simulink model "quadrotorsmodel1"  (R2025b)
settings: Solver=FixedStepAuto  StartTime=0.0  StopTime=SimulationTime  FixedStep=timestep  RelTol=1e-3
values from neighbouring files (symbols this model uses):
  g = 9.81    [TESA_Workspace1.m]    (also in TESA_Workspace2.m)
  I = eye(3,3)    [TESA_Workspace1.m]    (also in TESA_Workspace2.m)
  K = [1 1 1 1 ... (first row only)    [TESA_Workspace1.m]    (also in TESA_Workspace2.m)
  Kp = 1*Kp    [TESA_Workspace1.m]    (also in TESA_Workspace2.m)
  Kr = 1*Kr    [TESA_Workspace1.m]    (also in TESA_Workspace2.m)
  Kv = 1*Kv    [TESA_Workspace1.m]    (also in TESA_Workspace2.m)
  Kw = 1*Kw    [TESA_Workspace1.m]    (also in TESA_Workspace2.m)
  m = 4.34    [TESA_Workspace1.m]    (also in TESA_Workspace2.m)
settings Model: Creator=worap  LastModifiedBy=Sitasen
settings DataIOCC: ExternalInput=inputStructure  LoadExternalInput=on

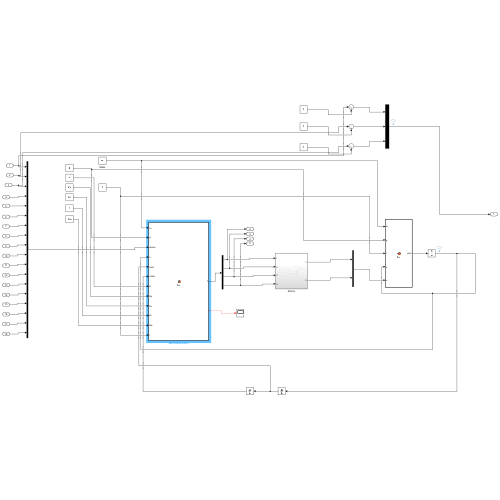
[thumbnail: Simulink's stored preview of the top-level diagram]
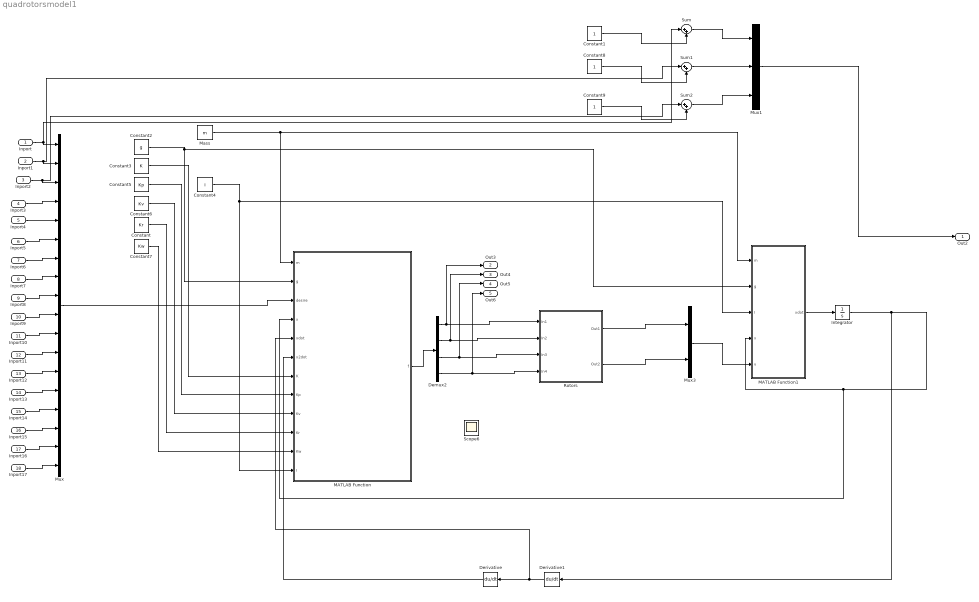
== system quadrotorsmodel1 ==
  Inport : Inport
  Inport1 : Inport  Port=2
  Inport2 : Inport  Port=3
  Inport3 : Inport  Port=4
  Inport4 : Inport  Port=5
  Inport5 : Inport  Port=6
  Inport6 : Inport  Port=7
  Inport7 : Inport  Port=8
  Inport8 : Inport  Port=9
  Inport9 : Inport  Port=10
  Inport10 : Inport  Port=11
  Inport11 : Inport  Port=12
  Inport12 : Inport  Port=13
  Inport13 : Inport  Port=14
  Inport14 : Inport  Port=15
  Inport15 : Inport  Port=16
  Inport16 : Inport  Port=17
  Inport17 : Inport  Port=18
  Constant : Constant  Value=Kr
  Constant1 : Constant
  Constant2 : Constant  Value=g
  Constant3 : Constant  Value=K
  Constant4 : Constant  Value=I
  Constant5 : Constant  Value=Kp
  Constant6 : Constant  Value=Kv
  Constant7 : Constant  Value=Kw
  Constant8 : Constant
  Constant9 : Constant
  Demux2 : Demux
  Derivative : Derivative
  Derivative1 : Derivative
  Integrator : Integrator  InitialCondition=[0;0;0;0;0;0;1;0;0;0;1;0;0;0;1;0;0;0]
  MATLAB Function : MATLAB Function  TreatAsAtomicUnit=on
  MATLAB Function1 : MATLAB Function  TreatAsAtomicUnit=on
  Mass : Constant  Value=m
  Mux : Mux  Inputs=18
  Mux1 : Mux  Inputs=3
  Mux3 : Mux  Inputs=2
  Rotors : Subsystem
  Scope6 : Scope
      settings: ActiveDisplayYMinimum=-0.10349  ActiveDisplayYMaximum=2.21622
  Sum : Sum  Inputs=|++
  Sum1 : Sum  Inputs=|++
  Sum2 : Sum  Inputs=|++
  Out2 : Outport
  Out3 : Outport  Port=2
  Out4 : Outport  Port=3
  Out5 : Outport  Port=4
  Out6 : Outport  Port=5
  wires:
  Mass/1 -> MATLAB Function1/1(m), MATLAB Function/1(m)
  Demux2/2 -> Out4/1, Rotors/2(In2)
  Rotors/1(Out1) -> Mux3/1
  Rotors/2(Out2) -> Mux3/2
  Demux2/3 -> Out5/1, Rotors/3(In3)
  Demux2/4 -> Out6/1, Rotors/4(In4)
  Constant4/1 -> MATLAB Function1/3(I), MATLAB Function/12(I)
  MATLAB Function/1(f) -> Demux2/1
  Demux2/1 -> Out3/1, Rotors/1(In1)
  Constant2/1 -> MATLAB Function1/2(g), MATLAB Function/2(g)
  Constant3/1 -> MATLAB Function/7(K)
  Constant5/1 -> MATLAB Function/8(Kp)
  Constant6/1 -> MATLAB Function/9(Kv)
  Constant7/1 -> MATLAB Function/11(Kw)
  Constant/1 -> MATLAB Function/10(Kr)
  ? -> Scope6/1
  Mux3/1 -> MATLAB Function1/5(u)
  MATLAB Function1/1(xdot) -> Integrator/1
  Integrator/1 -> MATLAB Function/4(x), MATLAB Function1/4(x), Derivative1/1
  Mux/1 -> MATLAB Function/3(desire)
  Inport17/1 -> Mux/18
  Inport16/1 -> Mux/17
  Inport15/1 -> Mux/16
  Inport14/1 -> Mux/15
  Inport13/1 -> Mux/14
  Inport12/1 -> Mux/13
  Inport11/1 -> Mux/12
  Inport10/1 -> Mux/11
  Inport9/1 -> Mux/10
  Inport8/1 -> Mux/9
  Inport7/1 -> Mux/8
  Inport6/1 -> Mux/7
  Inport5/1 -> Mux/6
  Inport4/1 -> Mux/5
  Inport3/1 -> Mux/4
  Inport2/1 -> Sum2/1, Mux/3
  Inport1/1 -> Sum1/1, Mux/2
  Inport/1 -> Sum/1, Mux/1
  Derivative/1 -> MATLAB Function/6(x2dot)
  Derivative1/1 -> MATLAB Function/5(xdot), Derivative/1
  Sum/1 -> Mux1/1
  Constant1/1 -> Sum/2
  Constant8/1 -> Sum1/2
  Constant9/1 -> Sum2/2
  Sum2/1 -> Mux1/3
  Sum1/1 -> Mux1/2
  Mux1/1 -> Out2/1

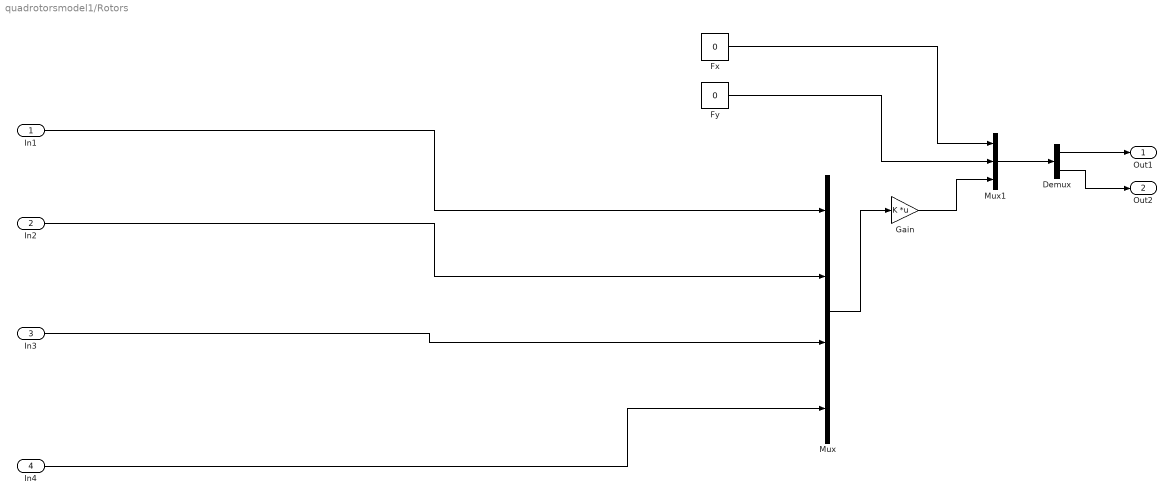
== system quadrotorsmodel1/Rotors ==
  In1 : Inport
  In2 : Inport  Port=2
  In3 : Inport  Port=3
  In4 : Inport  Port=4
  Demux : Demux  Outputs=2
  Fx : Constant  Value=0
  Fy : Constant  Value=0
  Gain : Gain  Gain=K  Multiplication=Matrix(K*u) (u vector)
  Mux : Mux
  Mux1 : Mux  Inputs=3
  Out1 : Outport
  Out2 : Outport  Port=2
  wires:
  Fx/1 -> Mux1/1
  Mux1/1 -> Demux/1
  Fy/1 -> Mux1/2
  Mux/1 -> Gain/1
  Gain/1 -> Mux1/3
  Demux/2 -> Out2/1
  Demux/1 -> Out1/1
  In1/1 -> Mux/1
  In2/1 -> Mux/2
  In3/1 -> Mux/3
  In4/1 -> Mux/4

== matlab function quadrotorsmodel1/MATLAB Function1 ==
  data: m input; g input; I input; x input; u input; xdot output
function xdot = fcn(m,g,I,x,u)

% extract the x-vextor
p = x(1:3,1);
v = x(4:6,1);
R = reshape(x(7:15,1),3,3);
omega = x(16:18,1);

%control signal
f = u(3,1);
M = u(4:6,1);

e3 = [0;0;1];


xdot = zeros(size(x));

xdot(1:3,1) = v;
xdot(4:6,1) = g*e3 - 1/m*f*R*e3;

Rdot = R*hatmap(omega);
xdot(7:15,1) = Rdot(:);

xdot(16:18,1) = I\(M - cross(omega,I*omega));

%ตัวสเต็ท  อย่าไปยุ่งกับอันสุดท้าย อันที่เป็นเลข 1 จารย์เอาไว้ตรวจ


end

== matlab function quadrotorsmodel1/MATLAB Function ==
  data: m input; g input; f output; desire input; x input; xdot input; x2dot input; K input; Kp input; Kv input; Kr input; Kw input; I input
function f   = fcn(m,g,desire,x,xdot,x2dot,K,Kp,Kv,Kr,Kw,I)

% persistent r2dot_prev;
% if isempty(r2dot_prev)
%     r2dot_prev = [0;0;0];
% end
tolerance = 1e-6;

vee_map = @(M) [M(3,2); M(1,3); M(2,1)];

xt = desire(1);
yt = desire(2) ;
zt = desire(3);

dxt = desire(4);
dyt = desire(5);
dzt = desire(6);

ddxt = desire(7);
ddyt = desire(8);
ddzt = desire(9);

dddxt = desire(10);
dddyt = desire(11);
dddzt = desire(12); 
ddddxt = desire(13);
ddddyt = desire(14);
ddddzt = desire(15);

psit = desire(16);
dpsit = desire(17);
ddpsit = desire(18);
r_current = x(1:3);
v_current = x(4:6);
R = reshape(x(7:15), 3, 3);
%d_R xdot
%dd_R x2dot
omega = x(16:18,1);
rd = [xt;yt;zt];
dv = [dxt;dyt;dzt];
da = [ddxt;ddyt;ddzt];
e3 = [0; 0; 1];
trajectory = [xt;yt;zt;psit];

%{
att = x(4:6);    % [phi; theta; psi]
phi = att(1);
theta = att(2);
psi = att(3);

c_phi = cos(phi); s_phi = sin(phi);
c_th = cos(theta); s_th = sin(theta);
c_psi = cos(psi); s_psi = sin(psi);

% --- 3. คำนวณเมทริกซ์การหมุนปัจจุบัน (R) ---
R = [c_psi*c_th, c_psi*s_th*s_phi - s_psi*c_phi, c_psi*s_th*c_phi + s_psi*s_phi;
     s_psi*c_th, s_psi*s_th*s_phi + c_psi*c_phi, s_psi*s_th*c_phi - c_psi*s_phi;
     -s_th,      c_th*s_phi,                    c_th*c_phi];

%}
%%ส่วน2
ex = r_current - rd;
ev = v_current - dv;

%ส่วน1
dd_xd = x2dot(1);

F_des_vec = -Kp * ex - Kv * ev + m * (g * e3 + dd_xd);
F_des_norm = norm(F_des_vec);




if F_des_norm < tolerance
    z_Bdes = e3;
else
    z_Bdes = F_des_vec / F_des_norm;
end


h = [cos(psit); sin(psit); 0];
y_Bdes_unnormalized = cross(z_Bdes, h);
y_Bdes_norm = norm(y_Bdes_unnormalized);
if y_Bdes_norm < tolerance
    % avoid singularity
    temp_vec = cross(e3, z_Bdes);
    if norm(temp_vec) < tolerance
        y_Bdes = [0;1;0];
    else
        y_Bdes = temp_vec / norm(temp_vec);
    end
else
    y_Bdes = y_Bdes_unnormalized / y_Bdes_norm;
end

x_Bdes = cross(y_Bdes, z_Bdes);

Rd = [x_Bdes, y_Bdes, z_Bdes];

 

f_total = F_des_vec' *R *e3;
% if f_total < 0
%     f_total = 0;
% end

eR_matrix = 0.5 * (Rd' * R - R' * Rd);
eR = vee_map(eR_matrix);

omega_d_des_body_frame = [0; 0; dpsit];
e_omega = omega - R' * Rd * omega_d_des_body_frame; 

M = -Kr * eR - Kw * e_omega + cross(omega, I * omega);
u = [f_total; M];
f = K \ u;

% f(f < 0) = 0;

display(f);


end
